simulink model "Simple_pendulum_system"  (R2023b)
settings: Solver=FixedStepAuto  StartTime=0.0  StopTime=10.0  FixedStep=0.01  RelTol=1e-3
settings Model: NumberOfSteps=2  Creator=Santhosh  LastModifiedBy=Santhosh

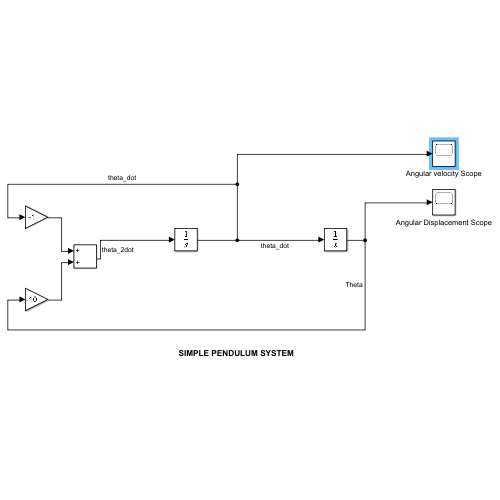
[thumbnail: Simulink's stored preview of the top-level diagram]
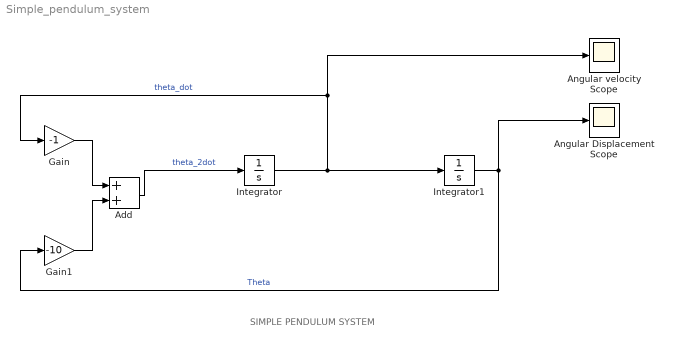
== system Simple_pendulum_system ==
  note: SIMPLE PENDULUM SYSTEM
  Add : Sum
  Angular Displacement Scope : Scope
  Angular velocity Scope : Scope
  Gain : Gain  Gain=-1
  Gain1 : Gain  Gain=-10
  Integrator : Integrator
  Integrator1 : Integrator  InitialCondition=0.1736481777
  wires:
  Integrator/1 -> Integrator1/1, Angular velocity Scope/1, Gain/1  "theta_dot"
  Integrator1/1 -> Gain1/1, Angular Displacement Scope/1  "Theta"
  Gain/1 -> Add/1
  Gain1/1 -> Add/2
  Add/1 -> Integrator/1  "theta_2dot"
